simulink model "PDFedbackControl2"  (R2017a)
settings: Solver=ode45  StartTime=0.0  StopTime=inf  MaxStep=0.001  RelTol=1e-3
values from neighbouring files (symbols this model uses):
  Kamp = 2.4    [lab5Script.m]
  Kpot = 1.6    [lab5Script.m]
  Ktach = 0.03    [lab5Script.m]
libraries: simulink x2
settings Model: Creator=maherna4  LastModifiedBy=maherna4

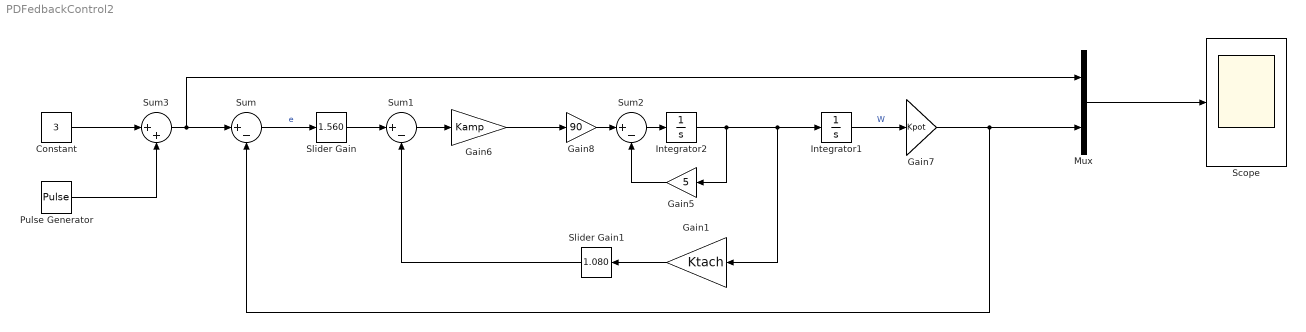
== system PDFedbackControl2 ==
  Constant : Constant  Value=3
  Gain1 : Gain  Gain=Ktach
  Gain5 : Gain  Gain=5
  Gain6 : Gain  Gain=Kamp
  Gain7 : Gain  Gain=Kpot
  Gain8 : Gain  Gain=90
  Integrator1 : Integrator
  Integrator2 : Integrator
  Mux : Mux  Inputs=2
  Pulse Generator : DiscretePulseGenerator  PulseType=Time based  Amplitude=2  PulseWidth=50
  Scope : Scope
  Slider Gain : simulink/Math Operations/Slider Gain  gain=1.560  low=0  high=2
  Slider Gain1 : simulink/Math Operations/Slider Gain  gain=1.080  low=0  high=2
  Sum : Sum  Inputs=|+-
  Sum1 : Sum  Inputs=|+-
  Sum2 : Sum  Inputs=|+-
  Sum3 : Sum  Inputs=|++
  wires:
  Slider Gain1/1 -> Sum1/2
  Sum/1 -> Slider Gain/1  "e"
  Integrator1/1 -> Gain7/1  "W"
  Gain7/1 -> Sum/2, Mux/2
  Gain1/1 -> Slider Gain1/1
  Sum1/1 -> Gain6/1
  Sum2/1 -> Integrator2/1
  Integrator2/1 -> Gain1/1, Integrator1/1, Gain5/1
  Gain5/1 -> Sum2/2
  Gain8/1 -> Sum2/1
  Gain6/1 -> Gain8/1
  Mux/1 -> Scope/1
  Constant/1 -> Sum3/1
  Pulse Generator/1 -> Sum3/2
  Sum3/1 -> Mux/1, Sum/1
  Slider Gain/1 -> Sum1/1
